simulink model "fedder"  (R2021b)
settings: Solver=FixedStepAuto  StartTime=0.0  StopTime=50.0  FixedStep=0.00000001  MaxStep=1.0  MinStep=1e-1  RelTol=1e-3
settings Model: SimulationMode=accelerator  Creator=Xavier  LastModifiedBy=Xavier
settings HardwareCC: ProdHWDeviceType=AMD->x86-64 (Windows64)

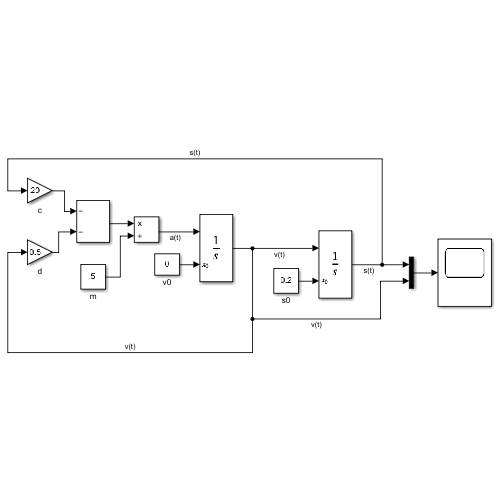
[thumbnail: Simulink's stored preview of the top-level diagram]
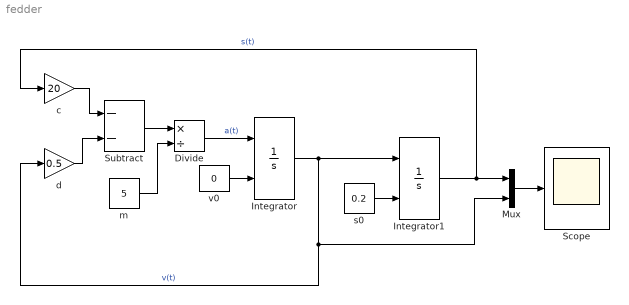
== system fedder ==
  Divide : Product  Inputs=*/
  Integrator : Integrator  InitialConditionSource=external
  Integrator1 : Integrator  InitialConditionSource=external
  Mux : Mux  Inputs=2
  Scope : Scope
  Subtract : Sum  Inputs=--
  c : Gain  Gain=20
  d : Gain  Gain=0.5
  m : Constant  Value=5
  s0 : Constant  Value=0.2
  v0 : Constant  Value=0
  wires:
  Mux/1 -> Scope/1
  Integrator1/1 -> c/1, Mux/1  "s(t)"
  Integrator/1 -> Mux/2, d/1, Integrator1/1  "v(t)"
  v0/1 -> Integrator/2
  s0/1 -> Integrator1/2
  Divide/1 -> Integrator/1  "a(t)"
  d/1 -> Subtract/2
  Subtract/1 -> Divide/1
  m/1 -> Divide/2
  c/1 -> Subtract/1
